simulink model "sys_ctrl_obs_luenberger_lineal"  (Simulink 7.9)
settings: Solver=ode45  StartTime=0.0  StopTime=Tt  RelTol=1e-3
undefined symbols (not defined in the file): A11, A12, A21, A22, Ad, B1, B2, Bd, Cd, Dd, K, Knoise, L, max_alpha, max_dalpha, max_dtheta, max_theta, min_alpha, min_dalpha, min_dtheta, min_theta, Ts, x_0
settings Model: Creator=pdoren  LastModifiedBy=matias  CovModelRefEnable=off
settings SolverCC: ZeroCrossAlgorithm=Adaptive
settings DataIOCC: SaveFormat=StructureWithTime  SignalLoggingSaveFormat=Dataset
settings OptimizationCC: ExpressionDepthLimit=128
settings DebuggingCC: UnderspecifiedInitializationDetection=Simplified  MergeDetectMultiDrivingBlocksExec=error  SolverPrmCheckMsg=none  StateNameClashWarn=none
settings HardwareCC: ProdBitPerPointer=64  ProdLargestAtomicFloat=Float  ProdIntDivRoundTo=Zero  ProdEndianess=LittleEndian  ProdHWDeviceType=Specified
settings CodeAppCC: CustomSymbolStrType=$N$R$M_T
settings GRTTargetCC: CodeReplacementLibrary=C89/C90 (ANSI)  GeneratePreprocessorConditionals=Use local settings  CombineOutputUpdateFcns=off  GRTInterface=on

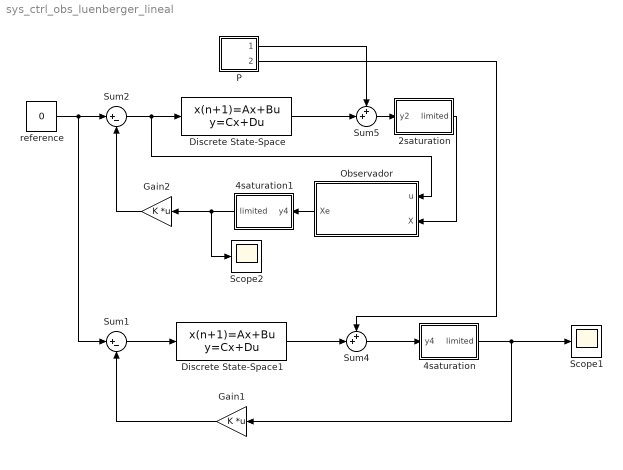
== system sys_ctrl_obs_luenberger_lineal ==
  2saturation : Subsystem
  4saturation : Subsystem
  4saturation1 : Subsystem
  Discrete State-Space : DiscreteStateSpace  A=Ad  B=Bd  C=Cd  D=Dd  X0=x_0  SampleTime=Ts
  Discrete State-Space1 : DiscreteStateSpace  A=Ad  B=Bd  C=eye(4)  D=zeros(4,1)  X0=x_0  SampleTime=Ts
  Gain1 : Gain  Gain=K  Multiplication=Matrix(K*u)
  Gain2 : Gain  Gain=K  Multiplication=Matrix(K*u)
  Observador : Subsystem
  P : Subsystem
  Scope1 : Scope
      settings: YMin=-2.0207  YMax=4.74305  SaveName=states_lineal_d
  Scope2 : Scope
      settings: YMin=-1246404085495577300000000000000000000000000000000000000000000000000000000000000000000000000000000000000000000000000000000000000000000000000000000000000000000000000000000000000000000000000000000000000000000000000000000000000000000000000000000000000000000000000000000000000000000000000000000000000000000000000.00000  YMax=4973481579999159400000000000000000000000000000000000000000000000000000000000000000000000000000000000000000000000000000000000000000000000000000000000000000000000000000000000000000000000000000000000000000000000000000000000000000000000000000000000000000000000000000000000000000000000000000000000000000000000000.00000  SaveName=states_lineal_d_obs
  Sum1 : Sum  Inputs=|+-
  Sum2 : Sum  Inputs=|+-
  Sum4 : Sum  Inputs=++|
  Sum5 : Sum  Inputs=++|
  reference : Constant  Value=0
  wires:
  Sum2/1 -> Discrete State-Space/1, Observador/1(u)
  Gain2/1 -> Sum2/2
  Discrete State-Space/1 -> Sum5/2
  reference/1 -> Sum1/1, Sum2/1
  Sum1/1 -> Discrete State-Space1/1
  Gain1/1 -> Sum1/2
  Discrete State-Space1/1 -> Sum4/2
  P/1(Noise2) -> Sum5/1
  P/2(Noise4) -> Sum4/1
  Sum5/1 -> 2saturation/1(y2)
  2saturation/1(limited) -> Observador/2(X)
  Sum4/1 -> 4saturation/1(y4)
  4saturation/1(limited) -> Scope1/1, Gain1/1
  Observador/1(Xe) -> 4saturation1/1(y4)
  4saturation1/1(limited) -> Gain2/1, Scope2/1

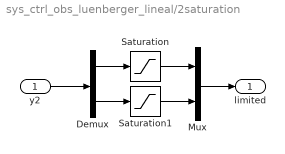
== system sys_ctrl_obs_luenberger_lineal/2saturation ==
  y2 : Inport
  Demux : Demux  Outputs=2
  Mux : Mux  Inputs=2
  Saturation : Saturate  UpperLimit=max_theta  LowerLimit=min_theta
  Saturation1 : Saturate  UpperLimit=max_dalpha  LowerLimit=min_dalpha
  limited : Outport
  wires:
  y2/1 -> Demux/1
  Demux/1 -> Saturation/1
  Demux/2 -> Saturation1/1
  Saturation/1 -> Mux/1
  Saturation1/1 -> Mux/2
  Mux/1 -> limited/1

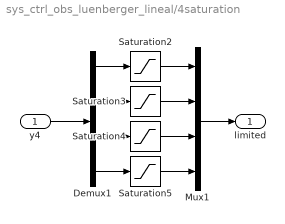
== system sys_ctrl_obs_luenberger_lineal/4saturation ==
  y4 : Inport
  Demux1 : Demux
  Mux1 : Mux
  Saturation2 : Saturate  UpperLimit=max_alpha  LowerLimit=min_alpha
  Saturation3 : Saturate  UpperLimit=max_theta  LowerLimit=min_theta
  Saturation4 : Saturate  UpperLimit=max_dalpha  LowerLimit=min_dalpha
  Saturation5 : Saturate  UpperLimit=max_dtheta  LowerLimit=min_dtheta
  limited : Outport
  wires:
  y4/1 -> Demux1/1
  Demux1/1 -> Saturation2/1
  Demux1/2 -> Saturation3/1
  Saturation2/1 -> Mux1/1
  Saturation3/1 -> Mux1/2
  Demux1/3 -> Saturation4/1
  Saturation4/1 -> Mux1/3
  Demux1/4 -> Saturation5/1
  Saturation5/1 -> Mux1/4
  Mux1/1 -> limited/1

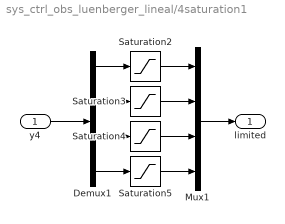
== system sys_ctrl_obs_luenberger_lineal/4saturation1 ==
  y4 : Inport
  Demux1 : Demux
  Mux1 : Mux
  Saturation2 : Saturate  UpperLimit=max_alpha  LowerLimit=min_alpha
  Saturation3 : Saturate  UpperLimit=max_theta  LowerLimit=min_theta
  Saturation4 : Saturate  UpperLimit=max_dalpha  LowerLimit=min_dalpha
  Saturation5 : Saturate  UpperLimit=max_dtheta  LowerLimit=min_dtheta
  limited : Outport
  wires:
  y4/1 -> Demux1/1
  Demux1/1 -> Saturation2/1
  Demux1/2 -> Saturation3/1
  Saturation2/1 -> Mux1/1
  Saturation3/1 -> Mux1/2
  Demux1/3 -> Saturation4/1
  Saturation4/1 -> Mux1/3
  Demux1/4 -> Saturation5/1
  Saturation5/1 -> Mux1/4
  Mux1/1 -> limited/1

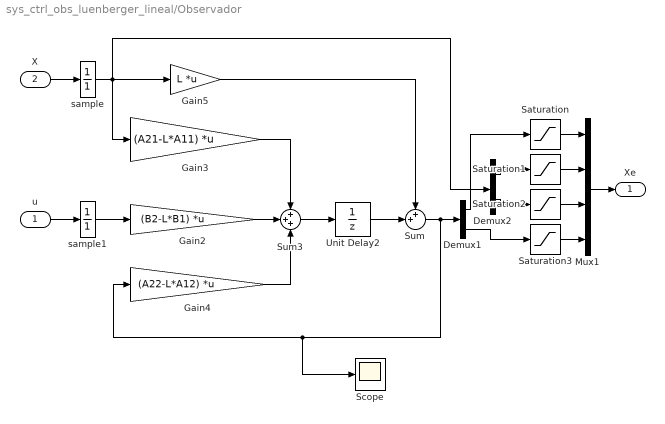
== system sys_ctrl_obs_luenberger_lineal/Observador ==
  u : Inport
  X : Inport  Port=2
  Demux1 : Demux  Outputs=2
  Demux2 : Demux  Outputs=2
  Gain2 : Gain  Gain=(B2-L*B1)  Multiplication=Matrix(K*u)
  Gain3 : Gain  Gain=(A21-L*A11)  Multiplication=Matrix(K*u)
  Gain4 : Gain  Gain=(A22-L*A12)  Multiplication=Matrix(K*u)
  Gain5 : Gain  Gain=L  Multiplication=Matrix(K*u)
  Mux1 : Mux
  Saturation : Saturate  UpperLimit=pi/4  LowerLimit=-pi/4
  Saturation1 : Saturate  UpperLimit=pi/4  LowerLimit=-pi/4
  Saturation2 : Saturate  UpperLimit=pi/2  LowerLimit=-pi/2
  Saturation3 : Saturate  UpperLimit=pi/2  LowerLimit=-pi/2
  Scope : Scope
      settings: YMin=-30.481  YMax=47.09183
  Sum : Sum  Inputs=++|
  Sum3 : Sum  Inputs=+++
  Unit Delay2 : UnitDelay  SampleTime=Ts
  sample : DiscreteTransferFcn  Denominator=[1]  SampleTime=Ts
  sample1 : DiscreteTransferFcn  Denominator=[1]  SampleTime=Ts
  Xe : Outport
  wires:
  Gain3/1 -> Sum3/1
  Gain4/1 -> Sum3/3
  Unit Delay2/1 -> Sum/2
  Sum3/1 -> Unit Delay2/1
  Gain2/1 -> Sum3/2
  Sum/1 -> Scope/1, Gain4/1, Demux1/1
  Gain5/1 -> Sum/1
  Mux1/1 -> Xe/1
  X/1 -> sample/1
  sample/1 -> Gain5/1, Demux2/1, Gain3/1
  u/1 -> sample1/1
  sample1/1 -> Gain2/1
  Saturation/1 -> Mux1/1
  Demux1/1 -> Saturation/1
  Saturation1/1 -> Mux1/2
  Demux2/1 -> Saturation1/1
  Saturation2/1 -> Mux1/3
  Demux2/2 -> Saturation2/1
  Saturation3/1 -> Mux1/4
  Demux1/2 -> Saturation3/1

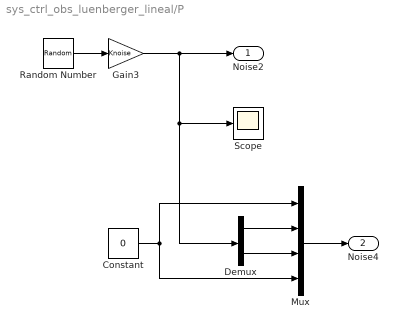
== system sys_ctrl_obs_luenberger_lineal/P ==
  Constant : Constant  Value=0
  Demux : Demux  Outputs=2
  Gain3 : Gain  Gain=Knoise
  Mux : Mux
  Random Number : RandomNumber  SampleTime=Ts
  Scope : Scope
      settings: YMin=-1.00000  YMax=1.00000
  Noise2 : Outport
  Noise4 : Outport  Port=2
  wires:
  Random Number/1 -> Gain3/1
  Gain3/1 -> Noise2/1, Demux/1, Scope/1
  Mux/1 -> Noise4/1
  Demux/1 -> Mux/2
  Demux/2 -> Mux/3
  Constant/1 -> Mux/4, Mux/1
